simulink model "lab10_pid_h1"  (R2023b)
settings: Solver=ode45  StartTime=0.0  StopTime=300.0  MaxStep=0.05  RelTol=1e-3
libraries: slpidlib x1, simulink x1
settings Model: Creator=insomnia  LastModifiedBy=insomnia

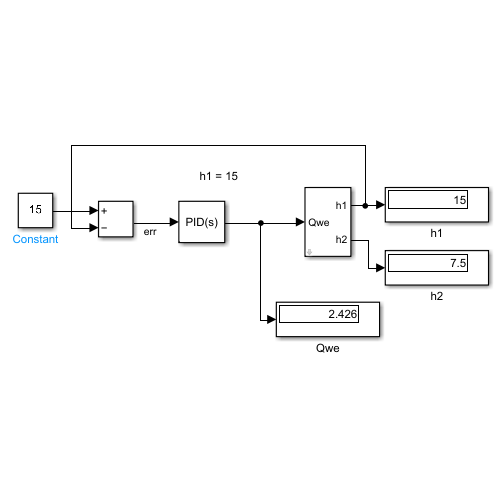
[thumbnail: Simulink's stored preview of the top-level diagram]
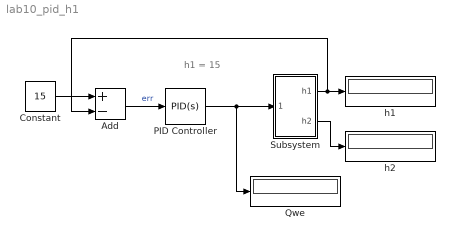
== system lab10_pid_h1 ==
  note: h1 = 15
  Add : Sum  Inputs=+-
  Constant : Constant  Value=15
  PID Controller : slpidlib/PID Controller  Controller=PID  Form=Parallel  TimeDomain=Continuous-time  UseExternalTs=off  SampleTime=-1  IntegratorMethod=Forward Euler  FilterMethod=Forward Euler  ControllerParametersSource=internal  P=1  I=1  UseKiTs=off  D=0  N=100  UseFilter=on  TunerSelectOption=Transfer Function Based (PID Tuner App)  InitialConditionSource=internal  InitialConditionForIntegrator=0  InitialConditionForFilter=0  DifferentiatorICPrevScaledInput=0  ExternalReset=none  TrackingMode=off  Kt=1  LimitOutput=off  SatLimitsSource=internal  UpperSaturationLimit=inf  LowerSaturationLimit=-inf  LinearizeAsGain=on  AntiWindupMode=none  Kb=1  LimitIntegrator=off  UpperIntegratorSaturationLimit=inf  LowerIntegratorSaturationLimit=-inf  POutMin=[]  POutMax=[]  IOutMin=[]  IOutMax=[]  DOutMin=[]  DOutMax=[]  NOutMin=[]  NOutMax=[]  SumOutMin=[]  SumOutMax=[]  SaturationOutMin=[]  SaturationOutMax=[]  PParamMin=[]  PParamMax=[]  IParamMin=[]  IParamMax=[]  DParamMin=[]  DParamMax=[]  NParamMin=[]  NParamMax=[]  KbParamMin=[]  KbParamMax=[]  KtParamMin=[]  KtParamMax=[]  KbOutMin=[]  KbOutMax=[]  KtOutMin=[]  KtOutMax=[]  IntegratorOutMin=[]  IntegratorOutMax=[]  FilterOutMin=[]  FilterOutMax=[]  SumI1OutMin=[]  SumI1OutMax=[]  SumI2OutMin=[]  SumI2OutMax=[]  SumI3OutMin=[]  SumI3OutMax=[]  SumI4OutMin=[]  SumI4OutMax=[]  SumDOutMin=[]  SumDOutMax=[]  DifferentiatorOutMin=[]  DifferentiatorOutMax=[]  FilterDiffOutCoefMin=[]  FilterDiffOutCoefMax=[]  ReciprocalOutMin=[]  ReciprocalOutMax=[]  SumDenOutMin=[]  SumDenOutMax=[]  SumNumOutMin=[]  SumNumOutMax=[]  DivideOutMin=[]  DivideOutMax=[]  UdiffTsProdOutMin=[]  UdiffTsProdOutMax=[]  NTsProdOutMin=[]  NTsProdOutMax=[]  UintegralTsProdOutMin=[]  UintegralTsProdOutMax=[]  UngainTsProdOutMin=[]  UngainTsProdOutMax=[]  ClampingZeroOutDataTypeStr=Inherit: Inherit via back propagation  ClampingZeroOutMin=[]  ClampingZeroOutMax=[]  FilterDenConstantOutDataTypeStr=Inherit: Inherit via back propagation  FilterDenConstantOutMin=[]  FilterDenConstantOutMax=[]  PCopyOutDataTypeStr=Inherit: Inherit via back propagation  PCopyOutMin=[]  PCopyOutMax=[]  NCopyOutDataTypeStr=Inherit: Inherit via back propagation  NCopyOutMin=[]  NCopyOutMax=[]  IntegratorContinuousStateAttributes=''  IntegratorStateMustResolveToSignalObject=off  IntegratorRTWStateStorageClass=Auto  FilterContinuousStateAttributes=''  FilterStateMustResolveToSignalObject=off  FilterRTWStateStorageClass=Auto  ParallelPVariant=InternalParameters  IdealPVariant=Disabled  IVariant=InternalParameters  DVariant=InternalParameters  IntegratorVariant=Continuous  SatVariant=Disabled  AWVariant=Passthrough  PCopyVariant=Disabled  TRVariant=Disabled  FdbkBlocksVariant=Forward  IdealPFdbkVariant=Disabled  SatFdbkVariant=Disabled  DerivativeFilterVariant=ContFilter  NVariant=InternalParameters  NCopyVariant=Disabled  FilterICVariant=InternalICsFilter  IntegratorICVariant=InternalICs  ExternalResetVariant=Disabled  TRSumVariant=Passthrough  SumFdbkVariant=Disabled  SumVariant=Sum_PID  TsampFilterVariant=InternalTs  TsampNgainVariant=Passthrough  TsampIntegralVariant=Disabled_SignalSpec  ExternalSaturationOutDataTypeStr=Inherit: Same as second input
  Qwe : Display
  Subsystem : Subsystem  mask{h1=4, h2=2, S1=1, S2=2, Swy1=0.2, Swy2=0.2, fi1=1, fi2=1, g=9.81, Qwe=2}
  h1 : Display
  h2 : Display
  wires:
  PID Controller/1 -> Subsystem/1(Qwe), Qwe/1
  Subsystem/1(h1) -> Add/2, h1/1
  Subsystem/2(h2) -> h2/1
  Add/1 -> PID Controller/1  "err"
  Constant/1 -> Add/1

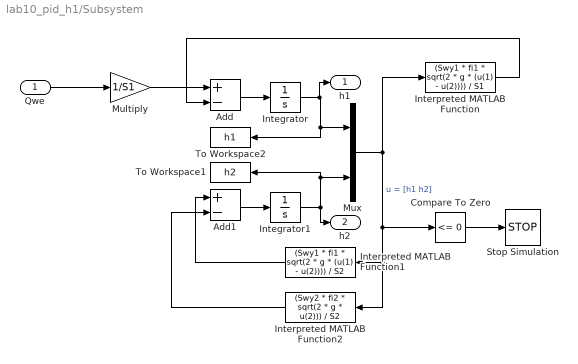
== system lab10_pid_h1/Subsystem ==
  Qwe : Inport
  Add : Sum  Inputs=+-
  Add1 : Sum  Inputs=+-
  Compare To Zero : simulink/Logic and Bit Operations/Compare To Zero  relop=<=  OutDataTypeStr=boolean
  Integrator : Integrator  InitialCondition=h1
  Integrator1 : Integrator  InitialCondition=h2
  Interpreted MATLAB Function : MATLABFcn  MATLABFcn=(Swy1 * fi1 * sqrt(2 * g * (u(1) - u(2)))) / S1
  Interpreted MATLAB Function1 : MATLABFcn  MATLABFcn=(Swy1 * fi1 * sqrt(2 * g * (u(1) - u(2)))) / S2
  Interpreted MATLAB Function2 : MATLABFcn  MATLABFcn=(Swy2 * fi2 * sqrt(2 * g * u(2))) / S2
  Multiply : Gain  Gain=1/S1
  Mux : Mux  Inputs=2
  Stop Simulation : Stop
  To Workspace1 : ToWorkspace  VariableName=h2  SampleTime=-1
  To Workspace2 : ToWorkspace  VariableName=h1  SampleTime=-1
  h1 : Outport
  h2 : Outport  Port=2
  wires:
  Multiply/1 -> Add/1
  Qwe/1 -> Multiply/1
  Add/1 -> Integrator/1
  Integrator/1 -> h1/1, To Workspace2/1, Mux/1
  Integrator1/1 -> h2/1, To Workspace1/1, Mux/2
  Add1/1 -> Integrator1/1
  Mux/1 -> Interpreted MATLAB Function/1, Compare To Zero/1, Interpreted MATLAB Function2/1, Interpreted MATLAB Function1/1  "u = [h1 h2]"
  Interpreted MATLAB Function/1 -> Add/2
  Interpreted MATLAB Function1/1 -> Add1/1
  Interpreted MATLAB Function2/1 -> Add1/2
  Compare To Zero/1 -> Stop Simulation/1
